simulink model "Lab_1_51"  (R2025b)
settings: Solver=ode45  StartTime=0.0  StopTime=10.0  FixedStep=0.75  MaxStep=1  MinStep=0  RelTol=1e-3
settings Model: Creator=james  LastModifiedBy=james
settings DataIOCC: ReturnWorkspaceOutputs=off

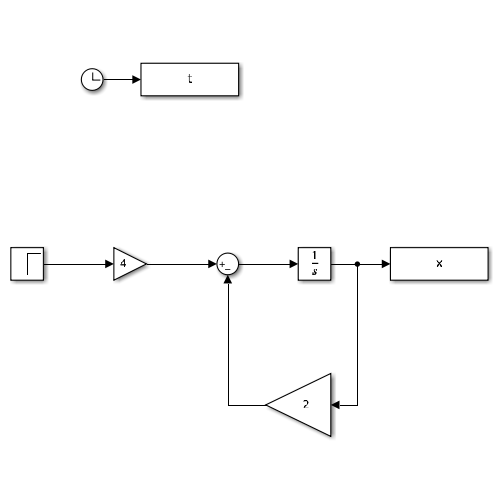
[thumbnail: Simulink's stored preview of the top-level diagram]
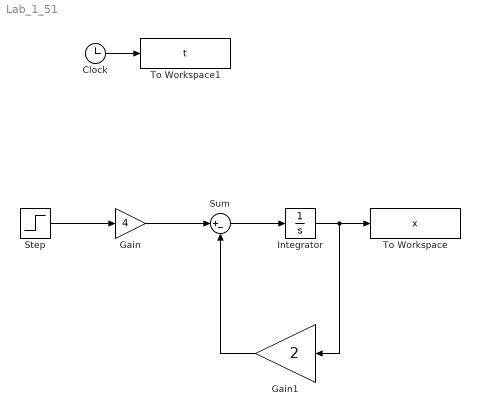
== system Lab_1_51 ==
  Clock : Clock
  Gain : Gain  Gain=4
  Gain1 : Gain  Gain=2
  Integrator : Integrator
  Step : Step  Time=0  SampleTime=0
  Sum : Sum  Inputs=|+-
  To Workspace : ToWorkspace  VariableName=x  SampleTime=-1
  To Workspace1 : ToWorkspace  VariableName=t  SampleTime=-1
  wires:
  Clock/1 -> To Workspace1/1
  Step/1 -> Gain/1
  Gain/1 -> Sum/1
  Sum/1 -> Integrator/1
  Integrator/1 -> Gain1/1, To Workspace/1
  Gain1/1 -> Sum/2
